simulink model "Pitch_Ap"  (Simulink 8.0)
settings: configuration reference "configSetObj_autopilot" (kept outside this file)
libraries: simulink x2, common_lib x1, aerolibconvert2 x1
settings Model: Creator=bpotter  LastModifiedBy=ssauvage  RecordCoverage=on  CovSaveName=covdata_pitchAP  CovMetricSettings=dcmtre  CovHTMLOptions=-aTS=1 -bRG=1 -bTC=1 -hTR=1 -nFC=0 -scm=1 -bcm=1  CovCumulativeVarName=covCumulativeData_pitchAP  CovCumulativeReport=on  CovReportOnPause=off
settings ConfigSet: SourceLocation=Base Workspace

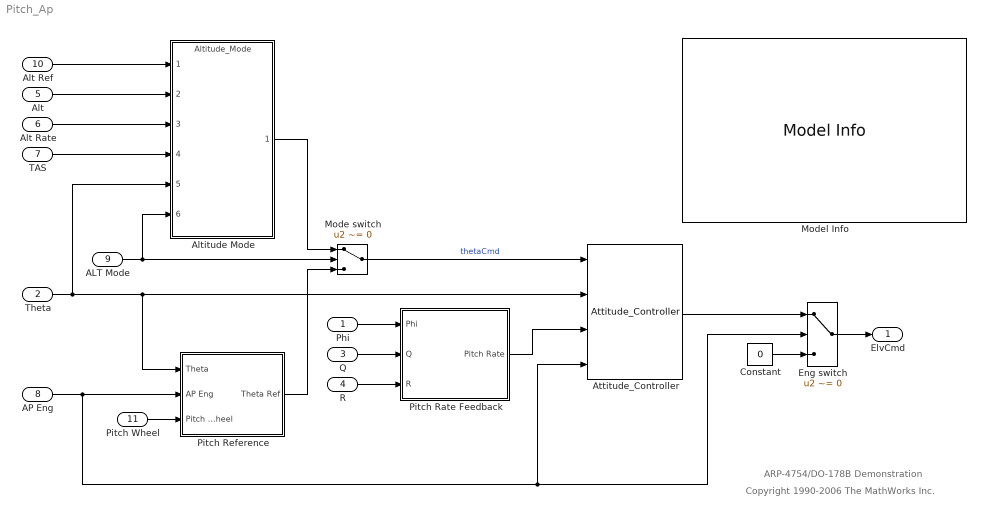
== system Pitch_Ap ==
  note: Copyright 1990-2006 The MathWorks Inc.
  note: ARP-4754/DO-178B Demonstration
  Phi : Inport  OutDataTypeStr=double  PortDimensions=1  SampleTime=1/40  Interpolate=off
  Theta : Inport  Port=2  OutDataTypeStr=double  PortDimensions=1  SampleTime=1/40  Interpolate=off
  Q : Inport  Port=3  OutDataTypeStr=double  PortDimensions=1  SampleTime=1/40  Interpolate=off
  R : Inport  Port=4  OutDataTypeStr=double  PortDimensions=1  SampleTime=1/40  Interpolate=off
  Alt : Inport  Port=5  OutDataTypeStr=double  PortDimensions=1  SampleTime=1/40  Interpolate=off
  Alt Rate : Inport  Port=6  OutDataTypeStr=double  PortDimensions=1  SampleTime=1/40  Interpolate=off
  TAS : Inport  Port=7  OutDataTypeStr=double  PortDimensions=1  SampleTime=1/40  Interpolate=off
  AP Eng : Inport  Port=8  OutDataTypeStr=boolean  PortDimensions=1  SampleTime=1/40  Interpolate=off
  ALT Mode : Inport  Port=9  OutDataTypeStr=boolean  PortDimensions=1  SampleTime=1/40  Interpolate=off
  Alt Ref : Inport  Port=10  OutDataTypeStr=double  PortDimensions=1  SampleTime=1/40  Interpolate=off
  "Pitch Wheel " : Inport  Port=11  OutDataTypeStr=double  PortDimensions=1  SampleTime=1/40  Interpolate=off
  Altitude Mode : ModelReference  ModelNameDialog=Altitude_Mode  SimulationMode=Normal  ModelReferenceVersion=1.84  CopyOfModelName=Altitude_Mode  DefaultDataLogging=off
  Attitude_Controller : common_lib/Attitude_Controller  dispGain=1  dispLim=20  rateGain=3  rateLim=3  intGain=1  intLim=5  cmdLim=20
  Constant : Constant  Value=0  OutDataTypeStr=double
  Eng switch : Switch  Criteria=u2 ~= 0
  Mode switch : Switch  Criteria=u2 ~= 0
  Model Info : simulink/Model-Wide Utilities/Model Info  InitialBlockCM=None  BlockCM=None  Frame=on  DisplayStringWithTags=|  HorizontalTextAlignment=Left  LeftAlignmentValue=0.02  SourceBlockDiagram=Pitch_Ap  TagMaxNumber=20
      | Pitch Autopilot
      | Author: %<LastModifiedBy>
      | Date: %<LastModificationDate>
      | Model Version: %<ModelVersion>
      | DO-178B Software Lifecycle Data:
      |   11.9 Software Requirements Data
      |   11.10 Design Description
      | DO-178B Objectives:
      |   5.1.1a High Level Requirements are Developed
      |   5.1.1b Derived High Level Requirements are Developed
      |   5.2.1a Low Level Requirements are Developed
      |   5.2.1a Software Architecture is Developed
      |   5.2.1b  Derived Low Level Requirements are Developed
  Pitch Rate Feedback : Subsystem  TreatAsAtomicUnit=on
      settings: RTWSystemCode=Inline
  Pitch Reference : Subsystem  TreatAsAtomicUnit=on
      settings: RTWSystemCode=Inline
  ElvCmd : Outport  OutDataTypeStr=double  PortDimensions=1  SampleTime=1/40
  wires:
  Alt Ref/1 -> Altitude Mode/1
  Theta/1 -> Pitch Reference/1(Theta), Attitude_Controller/2, Altitude Mode/5
  Q/1 -> Pitch Rate Feedback/2(Q)
  Alt/1 -> Altitude Mode/2
  Alt Rate/1 -> Altitude Mode/3
  Mode switch/1 -> Attitude_Controller/1  "thetaCmd"
  ALT Mode/1 -> Mode switch/2, Altitude Mode/6
  Altitude Mode/1 -> Mode switch/1
  AP Eng/1 -> Eng switch/2, Attitude_Controller/4, Pitch Reference/2(AP Eng)
  Eng switch/1 -> ElvCmd/1
  Constant/1 -> Eng switch/3
  Phi/1 -> Pitch Rate Feedback/1(Phi)
  R/1 -> Pitch Rate Feedback/3(R)
  TAS/1 -> Altitude Mode/4
  Pitch Reference/1(Theta Ref) -> Mode switch/3
  "Pitch Wheel "/1 -> Pitch Reference/3(Pitch Wheel)
  Pitch Rate Feedback/1(Pitch Rate) -> Attitude_Controller/3
  Attitude_Controller/1 -> Eng switch/1

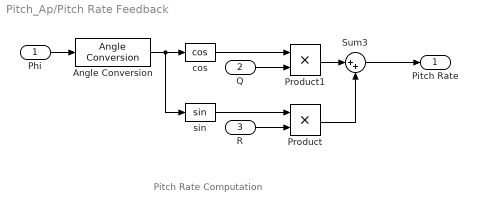
== system Pitch_Ap/Pitch Rate Feedback ==
  note: Pitch Rate Computation
  Phi : Inport
  Q : Inport  Port=2
  R : Inport  Port=3
  Angle Conversion : aerolibconvert2/Angle Conversion  IU=deg  OU=rad
  Product : Product  RndMeth=Zero
  Product1 : Product  RndMeth=Zero
  Sum3 : Sum  Inputs=|++
  cos : Trigonometry  Operator=cos  OutputSignalType=real
  sin : Trigonometry  OutputSignalType=real
  Pitch Rate : Outport
  wires:
  Phi/1 -> Angle Conversion/1
  Product/1 -> Sum3/2
  sin/1 -> Product/1
  R/1 -> Product/2
  Angle Conversion/1 -> sin/1, cos/1
  Product1/1 -> Sum3/1
  cos/1 -> Product1/1
  Q/1 -> Product1/2
  Sum3/1 -> Pitch Rate/1

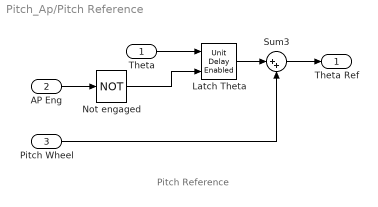
== system Pitch_Ap/Pitch Reference ==
  note: Pitch Reference
  Theta : Inport
  AP Eng : Inport  Port=2
  Pitch Wheel : Inport  Port=3
  Latch Theta : simulink/Additional Math & Discrete/Additional Discrete/Unit Delay Enabled  vinit=0.0  tsamp=1/40
  Not engaged : Logic  Operator=NOT  IconShape=distinctive  AllPortsSameDT=off  OutDataTypeStr=boolean
  Sum3 : Sum  Inputs=|++
  Theta Ref : Outport
  wires:
  Not engaged/1 -> Latch Theta/2
  Latch Theta/1 -> Sum3/1
  Theta/1 -> Latch Theta/1
  AP Eng/1 -> Not engaged/1
  Sum3/1 -> Theta Ref/1
  Pitch Wheel/1 -> Sum3/2
